simulink model "UAV_NL_Aug"  (Simulink 7.8)
settings: Solver=ode3  StartTime=0.0  StopTime=40  RelTol=1e-3
values from neighbouring files (symbols this model uses):
  k_opt = 0.001*t    [SAS_dampers.m]
  kp = z_opt(z)    [SAS_dampers.m]
  kr = z_opt(z)    [SAS_dampers.m]
  pitch_input = 0    [SAS_dampers.m]
  roll_input = 1    [SAS_dampers.m]
  yaw_input = 1    [SAS_dampers.m]
undefined symbols (not defined in the file or in its folder): sigbuilder_block
libraries: simulink_extras x14, Actuator_Lib x2, simulink x2, NonlinearModel_Lib x1, Sensors_Lib x1, cstblocks x1
settings Model: Creator=david  LastModifiedBy=david

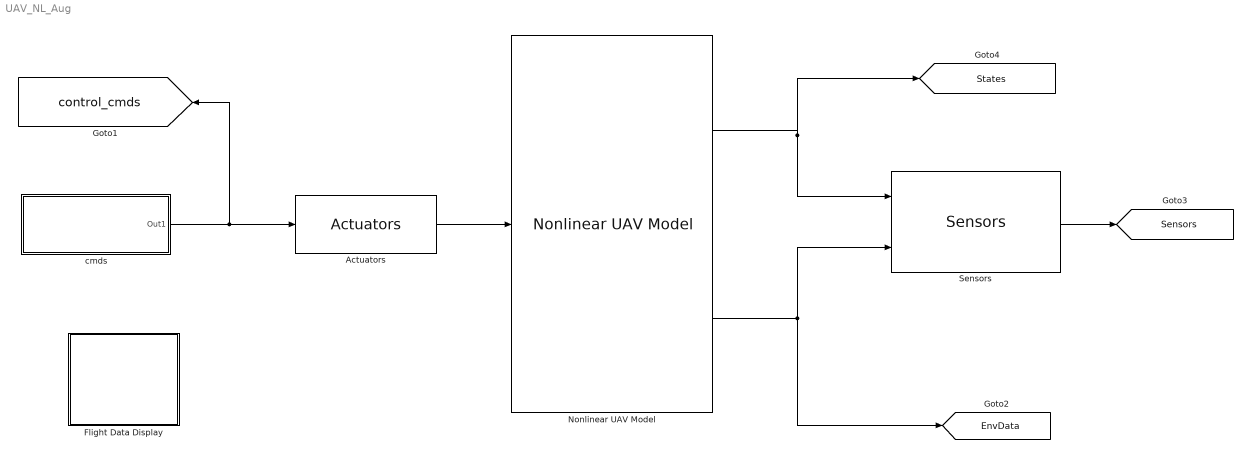
== system UAV_NL_Aug ==
  Actuators : Actuator_Lib/Actuators
  Flight Data Display : Subsystem
      mask Display:
      | x = 0:.1:2*pi;
      | plot(x,sin(x)+rand(size(x))*.5)
  Nonlinear UAV Model : NonlinearModel_Lib/Nonlinear UAV Model
  Sensors : Sensors_Lib/Sensors
  cmds : Subsystem
  tag scope: EnvData=global, Sensors=global, States=global, control_cmds=global
  wires:
  cmds/1(Out1) -> Actuators/1, [control_cmds]
  Actuators/1 -> Nonlinear UAV Model/1
  Nonlinear UAV Model/1 -> Sensors/1, [States]
  Nonlinear UAV Model/2 -> Sensors/2, [EnvData]
  Sensors/1 -> [Sensors]

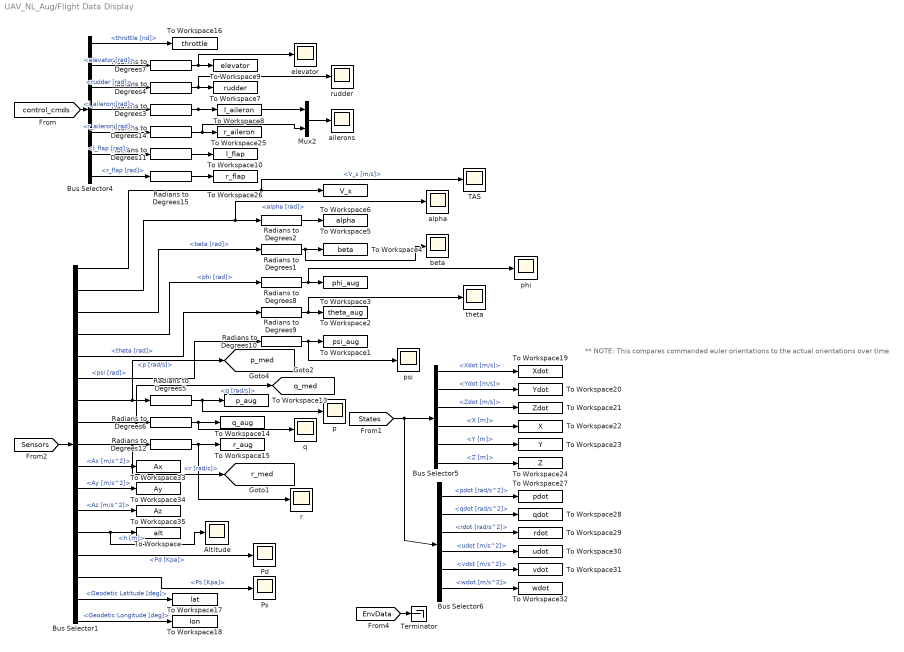
== system UAV_NL_Aug/Flight Data Display ==
  note: ** NOTE: This compares commanded euler orientations to the actual orientations over time
  Altitude : Scope
      settings: TimeRange=60  YMin=75  YMax=115  SaveName=ScopeData10
  Bus Selector1 : BusSelector  OutputSignals=V_s [m/s],alpha [rad],beta [rad],phi [rad],theta [rad],psi [rad],p [rad/s],q [rad/s],r [rad/s],Ax [m/s^2],Ay [m/s^2],Az [m/s^2],h [m],Pd [Kpa],Ps [Kpa],Geodetic Latitude [deg],Geodetic Longitude [deg]
  Bus Selector4 : BusSelector  OutputSignals=throttle [nd],elevator [rad],rudder [rad],l_aileron [rad],r_aileron [rad],l_flap [rad],r_flap [rad]
  Bus Selector5 : BusSelector  OutputSignals=V_e [m/s].Xdot [m/s],V_e [m/s].Ydot [m/s],V_e [m/s].Zdot [m/s],X_e [m].X [m],X_e [m].Y [m],X_e [m].Z [m]
  Bus Selector6 : BusSelector  OutputSignals=AngAccel [rad/s^2].pdot [rad/s^2],AngAccel [rad/s^2].qdot [rad/s^2],AngAccel [rad/s^2].rdot [rad/s^2],A_b [m/s^2].udot [m/s^2],A_b [m/s^2].vdot [m/s^2],A_b [m/s^2].wdot [m/s^2]
  Mux2 : Mux  Inputs=2
  Pd : Scope
      settings: TimeRange=25  YMin=0.14  YMax=0.2  SaveName=ScopeData5
  Ps : Scope
      settings: TimeRange=25  YMin=100.45  YMax=100.52  SaveName=ScopeData6
  Radians to Degrees{1..12,14..15} (14 alike) : simulink_extras/Transformations/Radians to Degrees
  TAS : Scope
      settings: TimeRange=45  YMin=14  YMax=19  SaveName=ScopeData3
  Terminator : Terminator
  To Workspace : ToWorkspace  VariableName=alt  SampleTime=-1  SaveFormat=Array
  To Workspace1 : ToWorkspace  VariableName=psi_aug  SampleTime=-1  SaveFormat=Array
  To Workspace10 : ToWorkspace  VariableName=l_flap  SampleTime=-1  SaveFormat=Array
  To Workspace13 : ToWorkspace  VariableName=p_aug  SampleTime=-1  SaveFormat=Array
  To Workspace14 : ToWorkspace  VariableName=q_aug  SampleTime=-1  SaveFormat=Array
  To Workspace15 : ToWorkspace  VariableName=r_aug  SampleTime=-1  SaveFormat=Array
  To Workspace16 : ToWorkspace  VariableName=throttle  SampleTime=-1  SaveFormat=Array
  To Workspace17 : ToWorkspace  VariableName=lat  SampleTime=-1  SaveFormat=Array
  To Workspace18 : ToWorkspace  VariableName=lon  SampleTime=-1  SaveFormat=Array
  To Workspace19 : ToWorkspace  VariableName=Xdot  SampleTime=-1  SaveFormat=Array
  To Workspace2 : ToWorkspace  VariableName=theta_aug  SampleTime=-1  SaveFormat=Array
  To Workspace20 : ToWorkspace  VariableName=Ydot  SampleTime=-1  SaveFormat=Array
  To Workspace21 : ToWorkspace  VariableName=Zdot  SampleTime=-1  SaveFormat=Array
  To Workspace22 : ToWorkspace  VariableName=X  SampleTime=-1  SaveFormat=Array
  To Workspace23 : ToWorkspace  VariableName=Y  SampleTime=-1  SaveFormat=Array
  To Workspace24 : ToWorkspace  VariableName=Z  SampleTime=-1  SaveFormat=Array
  To Workspace25 : ToWorkspace  VariableName=r_aileron  SampleTime=-1  SaveFormat=Array
  To Workspace26 : ToWorkspace  VariableName=r_flap  SampleTime=-1  SaveFormat=Array
  To Workspace27 : ToWorkspace  VariableName=pdot  SampleTime=-1  SaveFormat=Array
  To Workspace28 : ToWorkspace  VariableName=qdot  SampleTime=-1  SaveFormat=Array
  To Workspace29 : ToWorkspace  VariableName=rdot  SampleTime=-1  SaveFormat=Array
  To Workspace3 : ToWorkspace  VariableName=phi_aug  SampleTime=-1  SaveFormat=Array
  To Workspace30 : ToWorkspace  VariableName=udot  SampleTime=-1  SaveFormat=Array
  To Workspace31 : ToWorkspace  VariableName=vdot  SampleTime=-1  SaveFormat=Array
  To Workspace32 : ToWorkspace  VariableName=wdot  SampleTime=-1  SaveFormat=Array
  To Workspace33 : ToWorkspace  VariableName=Ax  SampleTime=-1  SaveFormat=Array
  To Workspace34 : ToWorkspace  VariableName=Ay  SampleTime=-1  SaveFormat=Array
  To Workspace35 : ToWorkspace  VariableName=Az  SampleTime=-1  SaveFormat=Array
  To Workspace4 : ToWorkspace  VariableName=beta  SampleTime=-1  SaveFormat=Array
  To Workspace5 : ToWorkspace  VariableName=alpha  SampleTime=-1  SaveFormat=Array
  To Workspace6 : ToWorkspace  VariableName=V_s  SampleTime=-1  SaveFormat=Array
  To Workspace7 : ToWorkspace  VariableName=rudder  SampleTime=-1  SaveFormat=Array
  To Workspace8 : ToWorkspace  VariableName=l_aileron  SampleTime=-1  SaveFormat=Array
  To Workspace9 : ToWorkspace  VariableName=elevator  SampleTime=-1  SaveFormat=Array
  ailerons : Scope
      settings: TimeRange=15  YMin=-0.6  YMax=0.6  SaveName=ScopeData2
  alpha : Scope
      settings: TimeRange=25  YMin=0.035  YMax=0.08  SaveName=ScopeData7
  beta : Scope
      settings: TimeRange=25  YMin=-0.06  YMax=0.06  SaveName=ScopeData11
  elevator : Scope
      settings: TimeRange=15  YMin=-5.78087  YMax=-5.23031
  p : Scope
      settings: TimeRange=45  YMin=-60  YMax=30  SaveName=ScopeData8
  phi : Scope
      settings: TimeRange=45  YMin=14  YMax=19  SaveName=ScopeData12
  psi : Scope
      settings: TimeRange=25  YMin=-0.06  YMax=0.06  SaveName=ScopeData14
  q : Scope
      settings: TimeRange=15  YMin=0.240133  YMax=0.265411  SaveName=ScopeData9
  r : Scope
      settings: TimeRange=45  YMin=-8  YMax=8
  rudder : Scope
      settings: TimeRange=45  YMin=-1.5  YMax=2  SaveName=ScopeData4
  theta : Scope
      settings: TimeRange=25  YMin=0.035  YMax=0.08  SaveName=ScopeData13
  tag scope: p_med=global, q_med=global, r_med=global
  wires:
  Bus Selector1/1 -> TAS/1, To Workspace6/1  "<V_s [m/s]>"
  Bus Selector1/2 -> Radians to Degrees2/1, alpha/1  "<alpha [rad]>"
  Radians to Degrees2/1 -> To Workspace5/1
  Bus Selector1/3 -> Radians to Degrees1/1  "<beta [rad]>"
  Radians to Degrees1/1 -> To Workspace4/1, beta/1
  Bus Selector1/4 -> Radians to Degrees8/1  "<phi [rad]>"
  Radians to Degrees8/1 -> To Workspace3/1, phi/1
  Bus Selector1/5 -> Radians to Degrees9/1  "<theta [rad]>"
  Radians to Degrees9/1 -> To Workspace2/1, theta/1
  Bus Selector1/6 -> Radians to Degrees10/1  "<psi [rad]>"
  Radians to Degrees10/1 -> To Workspace1/1, psi/1
  Radians to Degrees3/1 -> To Workspace8/1, Mux2/1
  Radians to Degrees7/1 -> To Workspace9/1, elevator/1
  Radians to Degrees4/1 -> To Workspace7/1, rudder/1
  Radians to Degrees11/1 -> To Workspace10/1
  Radians to Degrees5/1 -> To Workspace13/1, p/1
  Radians to Degrees6/1 -> To Workspace14/1, q/1
  Radians to Degrees12/1 -> To Workspace15/1, r/1
  [States] -> Bus Selector5/1, Bus Selector6/1
  Bus Selector5/1 -> To Workspace19/1  "<Xdot [m/s]>"
  Bus Selector5/2 -> To Workspace20/1  "<Ydot [m/s]>"
  Bus Selector5/3 -> To Workspace21/1  "<Zdot [m/s]>"
  Bus Selector5/4 -> To Workspace22/1  "<X [m]>"
  Bus Selector5/5 -> To Workspace23/1  "<Y [m]>"
  Bus Selector5/6 -> To Workspace24/1  "<Z [m]>"
  Bus Selector4/1 -> To Workspace16/1  "<throttle [nd]>"
  Bus Selector4/2 -> Radians to Degrees7/1  "<elevator [rad]>"
  Bus Selector4/3 -> Radians to Degrees4/1  "<rudder [rad]>"
  Bus Selector4/4 -> Radians to Degrees3/1  "<l_aileron [rad]>"
  Radians to Degrees14/1 -> To Workspace25/1, Mux2/2
  Bus Selector4/5 -> Radians to Degrees14/1  "<r_aileron [rad]>"
  Bus Selector4/6 -> Radians to Degrees11/1  "<l_flap [rad]>"
  Radians to Degrees15/1 -> To Workspace26/1
  Bus Selector4/7 -> Radians to Degrees15/1  "<r_flap [rad]>"
  Mux2/1 -> ailerons/1
  Bus Selector6/1 -> To Workspace27/1  "<pdot [rad/s^2]>"
  Bus Selector6/2 -> To Workspace28/1  "<qdot [rad/s^2]>"
  Bus Selector6/3 -> To Workspace29/1  "<rdot [rad/s^2]>"
  Bus Selector6/4 -> To Workspace30/1  "<udot [m/s^2]>"
  Bus Selector6/5 -> To Workspace31/1  "<vdot [m/s^2]>"
  Bus Selector6/6 -> To Workspace32/1  "<wdot [m/s^2]>"
  [control_cmds] -> Bus Selector4/1
  [Sensors] -> Bus Selector1/1
  Bus Selector1/7 -> Radians to Degrees5/1, [p_med]  "<p [rad/s]>"
  Bus Selector1/8 -> Radians to Degrees6/1, [q_med]  "<q [rad/s]>"
  Bus Selector1/9 -> Radians to Degrees12/1, [r_med]  "<r [rad/s]>"
  Bus Selector1/10 -> To Workspace33/1  "<Ax [m/s^2]>"
  Bus Selector1/11 -> To Workspace34/1  "<Ay [m/s^2]>"
  Bus Selector1/12 -> To Workspace35/1  "<Az [m/s^2]>"
  Bus Selector1/13 -> To Workspace/1, Altitude/1  "<h [m]>"
  Bus Selector1/14 -> Pd/1  "<Pd [Kpa]>"
  Bus Selector1/15 -> Ps/1  "<Ps [Kpa]>"
  Bus Selector1/16 -> To Workspace17/1  "<Geodetic Latitude [deg]>"
  Bus Selector1/17 -> To Workspace18/1  "<Geodetic Longitude [deg]>"
  [EnvData] -> Terminator/1

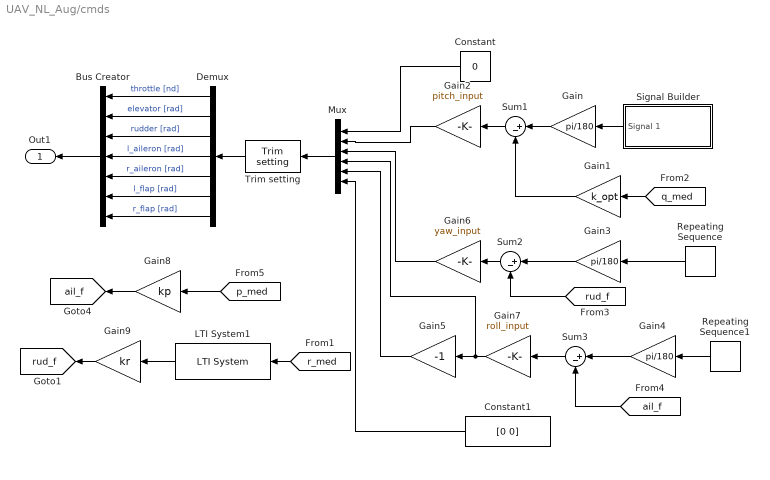
== system UAV_NL_Aug/cmds ==
  Bus Creator : BusCreator  Inputs=7
  Constant : Constant  Value=0
  Constant1 : Constant  Value=[0 0]
  Demux : Demux  Outputs=7
  Gain : Gain  Gain=pi/180
  Gain1 : Gain  Gain=k_opt
  Gain2 : Gain  Gain=pitch_input
  Gain3 : Gain  Gain=pi/180
  Gain4 : Gain  Gain=pi/180
  Gain5 : Gain  Gain=-1
  Gain6 : Gain  Gain=yaw_input
  Gain7 : Gain  Gain=roll_input
  Gain8 : Gain  Gain=kp
  Gain9 : Gain  Gain=kr
  LTI System1 : cstblocks/LTI System  sys=washout_filter  IC=[0]
  Mux : Mux  Inputs=6
  Repeating Sequence : simulink/Sources/Repeating Sequence  rep_seq_t=[0 2 2 3 3 4 4 100]  rep_seq_y=[0 0 10 10 -10 -10 0 0]
  Repeating Sequence1 : simulink/Sources/Repeating Sequence  rep_seq_t=[0 20 20 21 21 22 22 100]  rep_seq_y=[0 0 10 10 -10 -10 0 0]
  Signal Builder : Subsystem  Tag=STV Subsys  LoadFcn=sigbuilder_block('load');  StartFcn=sigbuilder_block('start');  StopFcn=sigbuilder_block('stop');  ClipboardFcn=sigbuilder_block('clipboard');  mask(Sigbuilder block){}
      mask help: Simulink:masks:SigbuilderBlock_MD
      mask init:
      | if ~strcmp(get_param(bdroot(gcbh),'SimulationStatus'),'stopped') tuvar = sigbuilder_block('maskInit'); end
      settings: CopyFcn=sigbuilder_block('copy');  DeleteFcn=sigbuilder_block('delete');  ModelCloseFcn=sigbuilder_block('modelClose');  PreSaveFcn=sigbuilder_block('preSave');  NameChangeFcn=sigbuilder_block('namechange');  OpenFcn=sigbuilder_block('open',[392.8 153.6 550.4 400 ]);  CloseFcn=sigbuilder_block('close');
      mask Display: plot(0, 0, 100, 100,[2, 2, 32, 32, 2], [68, 8, 8, 68, 68],[32, 2], [38, 38], [32, 19, 2],[53, 60, 44], [32, 17, 17, 2],[16, 16, 31, 31]);txt = getActiveGroup(gcbh);text(2, 100, txt,'verticalAlignment', 'top');
  Sum1 : Sum  Inputs=|+-
  Sum2 : Sum  Inputs=|+-
  Sum3 : Sum  Inputs=|+-
  "Trim setting " : Actuator_Lib/Trim setting 
  Out1 : Outport
  tag scope: ail_f=global, rud_f=global
  wires:
  Constant/1 -> Mux/1
  Demux/1 -> Bus Creator/1  "throttle [nd]"
  Demux/2 -> Bus Creator/2  "elevator [rad]"
  Demux/3 -> Bus Creator/3  "rudder [rad]"
  Demux/4 -> Bus Creator/4  "l_aileron [rad]"
  Demux/5 -> Bus Creator/5  "r_aileron [rad]"
  Demux/6 -> Bus Creator/6  "l_flap [rad]"
  Demux/7 -> Bus Creator/7  "r_flap [rad]"
  "Trim setting "/1 -> Demux/1
  Mux/1 -> "Trim setting "/1
  Bus Creator/1 -> Out1/1
  Signal Builder/1(Signal 1) -> Gain/1
  [q_med] -> Gain1/1
  Gain/1 -> Sum1/1
  Gain1/1 -> Sum1/2
  Sum1/1 -> Gain2/1
  Gain2/1 -> Mux/2
  Repeating Sequence1/1 -> Gain4/1
  Repeating Sequence/1 -> Gain3/1
  Gain4/1 -> Sum3/1
  [ail_f] -> Sum3/2
  Gain3/1 -> Sum2/1
  [rud_f] -> Sum2/2
  Sum2/1 -> Gain6/1
  Gain6/1 -> Mux/3
  Gain7/1 -> Gain5/1, Mux/4
  Sum3/1 -> Gain7/1
  Gain5/1 -> Mux/5
  Constant1/1 -> Mux/6
  [r_med] -> LTI System1/1
  Gain8/1 -> [ail_f]
  [p_med] -> Gain8/1
  LTI System1/1 -> Gain9/1
  Gain9/1 -> [rud_f]

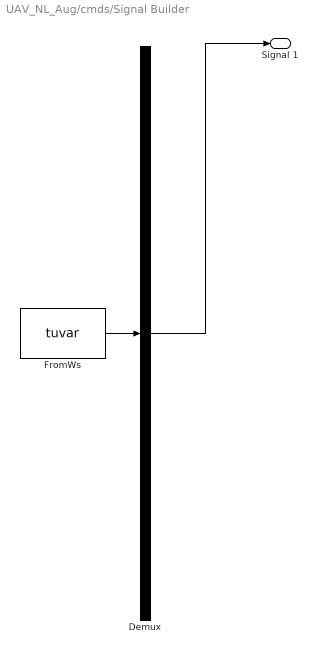
== system UAV_NL_Aug/cmds/Signal Builder ==
  Demux : Demux  Tag=STV Demux  Outputs=1
  FromWs : FromWorkspace  Tag=STV FromWs  VariableName=tuvar  SampleTime=0  SigBuilderData=DataTag0  VnvData=DataTag1
      SigBuilderData=|
      | common.afterFinalStr = 'Extrapolate'
      | common.sampleTime = 0
      | dataSet.timeRange = [0 12]
      | dataSet.name = 'Group 1'
      | sbobj.Groups.Name = 'Group 1'
      | sbobj.Groups.Signals.Name = 'Signal 1'
      | sbobj.Groups.Signals.XData = [0 3 3 4 4 5 5 12]
      | sbobj.Groups.Signals.YData = [0 0 10 10 -10 -10 0 0]
      | sbobj.Groups.TimeRange = [0 12]
  Signal 1 : Outport  Tag=STV Outport
  wires:
  Demux/1 -> Signal 1/1
  FromWs/1 -> Demux/1
